simulink model "cubesat_alg_dev_env"  (R2022a)
settings: Solver=FixedStepAuto  StartTime=0.0  StopTime=604800  FixedStep=0.5  MaxStep=1  MinStep=0.01  RelTol=1e-3
undefined symbols (not defined in the file or in its folder): km, s, WMM2020
libraries: aerolibutil x5, matrix_library x3, simulink_extras x1, vrlib x1, aerolibcelestial x1, aerolibgravity2 x1
settings Model: SimulationMode=accelerator  Creator=samuel  LastModifiedBy=samuel

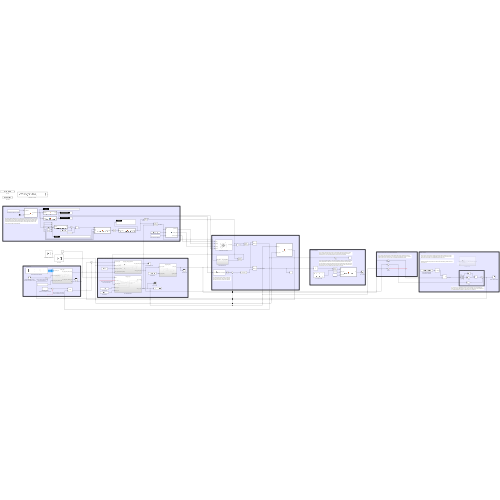
[thumbnail: Simulink's stored preview of the top-level diagram]
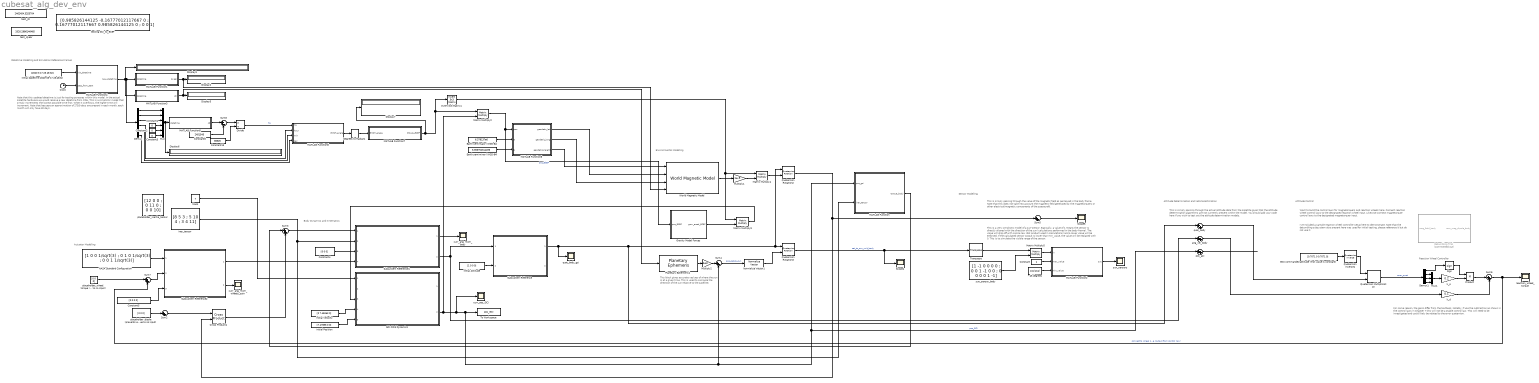
== system cubesat_alg_dev_env ==
  note: This block gives accurate vaslues of where the sun is at a given time. This is used to compute the direction of the sun relative to the satellite.
  note: For some reason, the gains differ from the textbook. Notably, if use the subtraction as shown in the control laws in Chapter 7 this will not be a stable control law. This will need to be investigated and could likely be related to the error quaternion.
  note: Reaction Wheel Controller
  note: I've included a sample reaction wheel controller setup here to demonstrate. Note that the detumbling subsystem also present here was used for initial testing, please reference it but do not use it.
  note: Want to build the control laws for magnetorquers and reaction wheels here. Connect reaction wheel control laws to the designated reaction wheel input. Likewise connect magnetorquer control laws to the designated magnetorquer input.
  note: Note that this updated datetime is just for testing purposes within this model. In the actual satellite hardware we would receive a new datetime from CDH. This is a simplistic model that simply increments the lowest possible time first. When it overflows, the higher time will increment. Note that becuase an approximation of 275/9 days are present in each month, each month will only have 30 days.
  note: This is simply passing through the value of the magnetic field as perceived in the body frame. Note that this does not take into account the magnetic field generated by the magnetorquers or other electrical/magnetic components of the spacecraft.
  note: This is a very simplistic model of a sun-sensor. Basically, a value of 1 means the sensor is directly aligned with the direction of the sun (calculations performed in the body-frame). The value will drop off with cosine law (dot product used in calculations) and a lower value will be enforced. If the calculated sensor output is lower than min_value, the value will be replaced with 0. This is to simulate the visible range of the sensor.
  note: This is simply passing through the actual atittude data from the satellite given that the attitude determination algorithms are not currently present within the model. You should add your code here if you wish to test out the attitude determination models.
  note: Datetime Modelling and Simulation Reference Frames
  note: Attitude Control
  note: Actuator Modelling
  note: Attitude Determination and Vehicle Estimation
  note: Sensor Modelling
  note: Environmental Modelling
  note: Body Dynamics and Kinematics
  Clock : Clock
  Constant : Constant
  Constant1 : Constant  Value=0
  Constant13 : Constant  Value=36525
  Constant2 : Constant  Value=0
  Constant3 : Constant  Value=0
  Constant4 : Constant  Value=[0 0 0]
  Constant5 : Constant  Value=[0 0 0 0]
  Constant6 : Constant  Value=2451545
  Cross Product1 : matrix_library/Cross Product
      settings: SourceProductBaseCode=SL
  Degrees to Radians : simulink_extras/Transformations/Degrees to Radians
  Demux : Demux  Outputs=6
  Demux1 : Demux
  Detumbling Trial : Subsystem  Commented=on
  Display{2..3,5..7} (5 alike) : Display
  Divide : Product  Inputs=*/
  Earth semimajor (WGS-84) : Constant  Value=6.378137e6
  Earth semiminor (WGS-84) : Constant  Value=6.3567523142e6
  GCI COG Dynamics : Subsystem  ReferencedSubsystem=cog_dyn_gci
  Gravity Model Forces : Subsystem
  Initial Attitude : Constant  Value=[1 0 0 0]
  Initial Datetime 2020-03-17 23:48:32 : Constant  Value=[2020 3 17 23 48 32]
  Initial Position : Constant  Value=[7.178e6 0 0]
  Initial Velocity : Constant  Value=[0 7.452e3 0]
  Invert 3x3 Matrix1 : aerolibutil/Invert  3x3 Matrix
  MATLAB Function : MATLAB Function  TreatAsAtomicUnit=on
  MATLAB Function1 : MATLAB Function  TreatAsAtomicUnit=on
  MATLAB Function2 : MATLAB Function  TreatAsAtomicUnit=on
  MATLAB Function3 : MATLAB Function  TreatAsAtomicUnit=on
  MATLAB Function4 : MATLAB Function  TreatAsAtomicUnit=on
  MATLAB Function5 : MATLAB Function  TreatAsAtomicUnit=on
  MATLAB Function6 : MATLAB Function  TreatAsAtomicUnit=on
  MATLAB Function7 : MATLAB Function  TreatAsAtomicUnit=on
  MATLAB Function8 : MATLAB Function  TreatAsAtomicUnit=on
  Mass : Constant  Value=7
  Matrix Multiply{2..5} (4 alike) : Product  Multiplication=Matrix(*)
  Multiply1 : Gain  Gain=1e-9
  Multiply2 : Gain  Gain=1e3
  Mux : Mux  Inputs=6
  Mux1 : Mux  Inputs=3
  NASA Standard Configuration : Constant  Value=[1 0 0 1/sqrt(3) ; 0 1 0 1/sqrt(3) ; 0 0 1 1/sqrt(3)]
  Normalize Vector1 : vrlib/Utilities/Normalize Vector  maxzero=0
  Planetary Ephemeris1 : aerolibcelestial/Planetary Ephemeris  kmflag=km,km/s  epochflag=Julian date  de=DE405  nCenter=Earth  nTarget=Sun  errorflag=Error  velflag=off
      settings: SourceProductBaseCode=AE
  Product : Product
  Quaternion Inverse1 : aerolibutil/Quaternion Inverse
  Quaternion Multiplication : aerolibutil/Quaternion Multiplication
  Quaternion Rotation2 : aerolibutil/Quaternion Rotation
  Quaternion Rotation3 : aerolibutil/Quaternion Rotation
  Scope4 : Scope
  Scope5 : Scope
  Sign : Signum
  Subsystem Reference : Subsystem  ReferencedSubsystem=quat_kin_body
  Subsystem Reference1 : Subsystem  ReferencedSubsystem=quat_dyn_body_w_wheels
  Subsystem Reference2 : Subsystem  ReferencedSubsystem=wheel_dyn
  Sum{2..3,5..7} (5 alike) : Sum  Inputs=|++
  Sum4 : Sum  Inputs=|+-
  Sum8 : Sum  Inputs=|+-
  To Workspace : ToWorkspace  VariableName=pos_GCI  SampleTime=-1
  Transpose : matrix_library/Transpose
      settings: SourceProductBaseCode=SL
  World Magnetic Model : aerolibgravity2/World Magnetic Model  model=WMM2020 (2020-2025)  customFile='WMM2020.COF'  units=Metric (MKS)  time_in=on  month=January  day=1  year=2020  action=Error  h_out=off  dec_out=off  inc_out=off  ti_out=off
      settings: SourceProductBaseCode=AE
  ang_vel_body : Sum  Inputs=|++
  curr_ang_mom_body : Scope
  curr_ang_mom_wheels_spin : Scope
  curr_pos_GCI : Scope
  iner_tensor : Constant  Value=[8 5 3 ; 5 10 4 ; 3 4 11]
  k_d : Gain  Gain=0.1
  k_p : Gain  Gain=0.2
  placeholder_dipole (prevents errors due to no input) : Constant  Value=[0 0 0]
  placeholder_inertia_tensor : Constant  Value=[12 0 0 ; 0 11 0 ; 0 0 10]
  placeholder_wheel_torque (prevents errors due to no input) : Constant  Value=[0 0 0]
  pos_gci : Sum  Inputs=|++
  quat_body : Sum  Inputs=|++
  quat_body_gci : Scope
  reaction_wheel_torque : Scope
  sun_sensor_body : Constant  Value=[1 -1 0 0 0 0 ; 0 0 1 -1 0 0 ; 0 0 0 0 1 -1]
  sun_sensors : Scope
  test commanded attitude (first value is constant) : Constant  Value=[0.7071 0 0.7071 0]
  test_JD : Constant  Value=2462454.3253704
  test_dyear : Constant  Value=2020.2986146465
  testing GCI_to_ECEF : Constant  Value=[0.985826144125 -0.16777012117667 0 ; 0.16777012117667 0.985826144125 0 ; 0 0 1]
  ~45 degrees : Constant  Value=cos(pi/4)
  wires:
  NASA Standard Configuration/1 -> Subsystem Reference2/1
  Initial Attitude/1 -> Subsystem Reference/2
  Constant5/1 -> Subsystem Reference2/3
  Mass/1 -> GCI COG Dynamics/1
  Initial Velocity/1 -> GCI COG Dynamics/4
  Initial Position/1 -> GCI COG Dynamics/5
  GCI COG Dynamics/2 -> To Workspace/1, pos_gci/1, MATLAB Function/1(pos_gci), Sum4/2, curr_pos_GCI/1, Matrix Multiply2/2  "pos_GCI"
  Sum7/1 -> Subsystem Reference2/2
  Subsystem Reference2/2 -> curr_ang_mom_wheels_spin/1
  Matrix Multiply2/1 -> MATLAB Function8/1(pos), Gravity Model Forces/1(pos_ECEF)  "pos_ECEF"
  MATLAB Function8/1(geodetic_lat) -> World Magnetic Model/2
  MATLAB Function8/2(geodetic_long) -> World Magnetic Model/3
  MATLAB Function8/3(geodetic_height) -> World Magnetic Model/1
  Gravity Model Forces/1(grav_accel_ECEF) -> Matrix Multiply3/2
  Invert 3x3 Matrix1/1 -> Matrix Multiply4/1, Matrix Multiply3/1
  Matrix Multiply3/1 -> GCI COG Dynamics/3
  iner_tensor/1 -> MATLAB Function/2(iner_tensor), Subsystem Reference1/2
  Constant4/1 -> Subsystem Reference1/3
  Subsystem Reference2/1 -> Subsystem Reference1/4
  Subsystem Reference1/1 -> curr_ang_mom_body/1
  Subsystem Reference1/2 -> ang_vel_body/1, Subsystem Reference/1
  World Magnetic Model/1 -> Multiply1/1
  Multiply1/1 -> Matrix Multiply4/2
  Matrix Multiply4/1 -> Quaternion Rotation2/2
  Subsystem Reference/1 -> Quaternion Rotation2/1, Quaternion Rotation3/1, quat_body/1, quat_body_gci/1
  placeholder_dipole (prevents errors due to no input)/1 -> Sum2/1
  ? -> Sum2/2  "connect to magnetic control dipole (output from magnetorquer model)"
  Quaternion Rotation2/1 -> Cross Product1/2, Sum5/1
  Sum2/1 -> Cross Product1/1
  Sum3/1 -> Subsystem Reference1/1
  Cross Product1/1 -> Sum3/2
  MATLAB Function/1(torque_body) -> Sum3/1
  Planetary Ephemeris1/1 -> Multiply2/1
  Normalize Vector1/1 -> Quaternion Rotation3/2
  Multiply2/1 -> Sum4/1
  Sum4/1 -> Normalize Vector1/1  "pos_sat_to_sun"
  sun_sensor_body/1 -> Matrix Multiply5/2
  Quaternion Rotation3/1 -> Scope4/1, Transpose/1  "sat_to_sun_unit_body"
  Transpose/1 -> Matrix Multiply5/1
  Sum5/1 -> Scope5/1
  Sum6/1 -> reaction_wheel_torque/1, Sum7/2  "connect to wheel control torque (output from control law)"
  placeholder_wheel_torque (prevents errors due to no input)/1 -> Sum7/1
  Matrix Multiply5/1 -> MATLAB Function2/1(in)
  Constant/1 -> MATLAB Function2/2(max_value)
  ~45 degrees/1 -> MATLAB Function2/3(min_value)
  MATLAB Function2/1(out) -> sun_sensors/1
  Clock/1 -> MATLAB Function4/2(secs_from_start)
  Initial Datetime 2020-03-17 23:48:32/1 -> MATLAB Function4/1(init_datetime)
  MATLAB Function4/1(new_datetime) -> Demux/1, MATLAB Function1/1(datetime), MATLAB Function3/1(datetime), Display3/1
  Demux/1 -> Mux/1
  Demux/2 -> Mux/2
  Demux/3 -> Mux/3
  Constant1/1 -> Mux/4
  Constant2/1 -> Mux/5
  Constant3/1 -> Mux/6
  Mux/1 -> Display6/1, MATLAB Function5/1(datetime)
  MATLAB Function5/1(JD) -> Sum8/1
  Constant6/1 -> Sum8/2
  Sum8/1 -> Divide/1
  Constant13/1 -> Divide/2
  Divide/1 -> MATLAB Function6/1(T0)  "T0"
  Demux/4 -> MATLAB Function6/2(hour)
  Demux/5 -> MATLAB Function6/3(min)
  Demux/6 -> MATLAB Function6/4(sec)
  MATLAB Function6/1(GMST_angle) -> Degrees to Radians/1
  Degrees to Radians/1 -> MATLAB Function7/1(GMST_angle)
  MATLAB Function7/1(GCI_to_ECEF) -> Matrix Multiply2/1, Invert 3x3 Matrix1/1, Display7/1
  MATLAB Function3/1(JD) -> Planetary Ephemeris1/1, Display5/1
  MATLAB Function1/1(dyear) -> World Magnetic Model/4, Display2/1
  ang_vel_body/1 -> k_d/1
  pos_gci/1 -> ?
  ? -> GCI COG Dynamics/2  "want to connect orbital disturbance forces to this block here"
  Demux1/2 -> Mux1/1
  Demux1/3 -> Mux1/2
  Demux1/4 -> Mux1/3
  Demux1/1 -> Sign/1
  Mux1/1 -> k_p/1
  k_p/1 -> Product/2
  Sign/1 -> Product/1
  Product/1 -> Sum6/1
  k_d/1 -> Sum6/2
  Quaternion Multiplication/1 -> Demux1/1  "error_quat"
  test commanded attitude (first value is constant)/1 -> Quaternion Inverse1/1
  Quaternion Inverse1/1 -> Quaternion Multiplication/1
  quat_body/1 -> Quaternion Multiplication/2
  Earth semiminor (WGS-84)/1 -> MATLAB Function8/3(b)
  Earth semimajor (WGS-84)/1 -> MATLAB Function8/2(a)

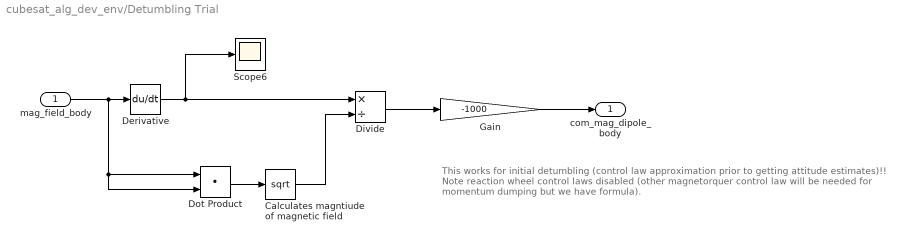
== system cubesat_alg_dev_env/Detumbling Trial ==
  note: This works for initial detumbling (control law approximation prior to getting attitude estimates)!! Note reaction wheel control laws disabled (other magnetorquer control law will be needed for momentum dumping but we have formula).
  mag_field_body : Inport
  Calculates magntiude of magnetic field : Sqrt
  Derivative : Derivative
  Divide : Product  Inputs=*/
  Dot Product : DotProduct  OutDataTypeStr=Inherit: Inherit via internal rule
  Gain : Gain  Gain=-1000
  Scope6 : Scope
  com_mag_dipole_body : Outport
  wires:
  Calculates magntiude of magnetic field/1 -> Divide/2
  Gain/1 -> com_mag_dipole_body/1
  Dot Product/1 -> Calculates magntiude of magnetic field/1
  Divide/1 -> Gain/1
  mag_field_body/1 -> Derivative/1, Dot Product/2, Dot Product/1
  Derivative/1 -> Divide/1, Scope6/1

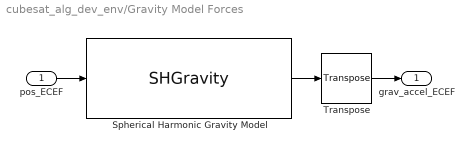
== system cubesat_alg_dev_env/Gravity Model Forces ==
  pos_ECEF : Inport
  Spherical Harmonic Gravity Model : SHGravity
  Transpose : matrix_library/Transpose
      settings: SourceProductBaseCode=SL
  grav_accel_ECEF : Outport
  wires:
  Spherical Harmonic Gravity Model/1 -> Transpose/1
  Transpose/1 -> grav_accel_ECEF/1
  pos_ECEF/1 -> Spherical Harmonic Gravity Model/1

== matlab function cubesat_alg_dev_env/MATLAB Function ==
  data: pos_gci input; torque_body output; iner_tensor input
function torque_body  = grav_grad_torque(pos_gci, iner_tensor)
    % mass of earth, grav constant
    m_e = 5.97219e24;
    G = 6.67430e-11;

    % grav param
    u = G*m_e;

    radius = norm(pos_gci);
    nadir_vec = -normalize(pos_gci);
    torque_body = cross(3*u/radius^3*nadir_vec, ...
        iner_tensor*nadir_vec);

== matlab function cubesat_alg_dev_env/MATLAB Function1 ==
  data: datetime input; dyear output
function dyear = dyear_from_datetime(datetime)

    % the datetime format is provided as a 6 value array
    % year, month, day, hour, minute, second

    % sequentially builds the decimal year

    % potentially we may want to use /61 for leap second days but this is
    % likely fine as our simulation just needs to perform regular datetime
    % updates for simple testing

    tot_mins = datetime(5) + datetime(6) / 60;
    tot_hours = datetime(4) + tot_mins / 60;
    tot_days = datetime(3) + tot_hours / 24;
    tot_months = datetime(2) + tot_days / (275/9); % average days in month across year
    tot_years = datetime(1) + tot_months / 12;

    dyear = tot_years;

== matlab function cubesat_alg_dev_env/MATLAB Function2 ==
  data: in input; out output; max_value input; min_value input
function out = zero_out_out_of_range(in, max_value, min_value)
    out = in;

    for i = 1:length(in)
        if out(i) < min_value || out(i) > max_value
            out(i) = 0;
        end
    end

== matlab function cubesat_alg_dev_env/MATLAB Function3 ==
  data: datetime input; JD output
function JD = calc_JD_from_datetime(datetime)

% the datetime format is provided as a 6 value array
% year, month, day, hour, minute, second

% calculates the Julian date (JD) from the datetime
JD = 1721013.5 + 367*datetime(1) - floor(7/4*(datetime(1) + ...
    floor((datetime(2) + 9)/12))) + floor(275/9*datetime(2)) + ...
    datetime(3) + (60*datetime(4) + datetime(5) + datetime(6)/60)/1440;

% note that seconds should be /61 for leap days but since we are using a
% testing environment we do not need to worry about this

% presumably in the navigation system of the actual satellite we may also
% not need to consider this as it would introduce a negligible error or we
% may need to have some special protocol with CDH to figure out a system

== matlab function cubesat_alg_dev_env/MATLAB Function4 ==
  data: init_datetime input; new_datetime output; secs_from_start input
function new_datetime  = datetime_upd(init_datetime, secs_from_start)

% the datetime format is provided as a 6 value array
% year, month, day, hour, minute, second

% initializes new datetime array
new_datetime = zeros(1, 6);

% adds the seconds from start of simulation to seconds
new_datetime(6) = init_datetime(6) + secs_from_start;

% computes the new seconds and minutes with carry over
new_datetime(5) = init_datetime(5) + floor(new_datetime(6) / 60);
new_datetime(6) = mod(new_datetime(6), 60);

% computes the new minutes and hours with carry over
new_datetime(4) = init_datetime(4) + floor(new_datetime(5) / 60);
new_datetime(5) = mod(new_datetime(5), 60);

% computes the new hours and days with carry over
new_datetime(3) = init_datetime(3) + floor(new_datetime(4) / 24);
new_datetime(4) = mod(new_datetime(4), 24);

% computes the new days and months with carry over
new_datetime(2) = init_datetime(2) + floor(new_datetime(3) / (275/9));

% NOTE: the floor here is specifically needed to prevent a recurring
% decimal from occurring here due to using an average number of days per
% month of 275/9 (this also caps days in a month to 30)
new_datetime(3) = floor(mod(new_datetime(3), (275/9)));

% computes the new months and years with carry over

% for calculations, shifts first month to 0
new_datetime(2) = new_datetime(2) - 1;

new_datetime(1) = init_datetime(1) + floor(new_datetime(2) / 12);

% done with calculations, restores first month to 1
new_datetime(2) = mod(new_datetime(2), 12) + 1;

end

== matlab function cubesat_alg_dev_env/MATLAB Function5 ==
  data: datetime input; JD output
function JD = calc_JD_from_datetime(datetime)

% the datetime format is provided as a 6 value array
% year, month, day, hour, minute, second

% calculates the Julian date (JD) from the datetime
JD = 1721013.5 + 367*datetime(1) - floor(7/4*(datetime(1) + ...
    floor((datetime(2) + 9)/12))) + floor(275/9*datetime(2)) + ...
    datetime(3) + (60*datetime(4) + datetime(5) + datetime(6)/60)/1440;

% note that seconds should be /61 for leap days but since we are using a
% testing environment we do not need to worry about this

% presumably in the navigation system of the actual satellite we may also
% not need to consider this as it would introduce a negligible error or we
% may need to have some special protocol with CDH to figure out a system

== matlab function cubesat_alg_dev_env/MATLAB Function6 ==
  data: T0 input; GMST_angle output; hour input; min input; sec input
function GMST_angle = calc_GMST_angle_from_T0(T0, hour, min, sec)

% calculates GMST_angle in units of seconds (longitudinal seconds)
GMST_angle = 24110.54841 + 8640184.812866 * T0 + 0.093104 * T0^2 ...
    - 6.2e-6 * T0^3 + 1.002737909350795 * (3600*hour + 60*min + sec);

% reduces to range of 0-86400
GMST_angle = mod(GMST_angle, 86400);

% converts to degrees (there are 240 longitudinal seconds in a degree)
GMST_angle = GMST_angle / 240;

== matlab function cubesat_alg_dev_env/MATLAB Function7 ==
  data: GMST_angle input; GCI_to_ECEF output
function GCI_to_ECEF = calc_GCI_to_ECEF_from_GMST_angle(GMST_angle)

% calculates the transformation matrix from GCI to ECEF
GCI_to_ECEF = [cos(GMST_angle) sin(GMST_angle) 0 ; ...
    -sin(GMST_angle) cos(GMST_angle) 0 ; 0 0 1];

== matlab function cubesat_alg_dev_env/MATLAB Function8 ==
  data: pos input; geodetic_lat output; a input; b input; geodetic_long output; geodetic_height output
function [geodetic_lat, geodetic_long, geodetic_height] = ...
    ECEF_coords_to_geodetic(pos, a, b)

    % converts from ECEF coordinates to geodetic coordinates

    x = pos(1);
    y = pos(2);
    z = pos(3);

    e2 = 1 - b^2 / a^2;
    eps2 = a^2 / b^2 - 1;
    rho = sqrt(x^2 + y^2);

    p = abs(z)/eps2;
    s = rho^2/(e2*eps2);
    q = p^2 - b^2 + s;

    u = p/sqrt(q);
    v = b^2*u^2/q;
    P=27*v*s/q;
    Q=(sqrt(P+1) + sqrt(P))^(2/3);

    t=(1+Q+1/Q)/6;
    c=sqrt(u^2-1+2*t);
    w=(c-u)/2;

    d=sign(z)*sqrt(q)*(w+sqrt(t^2+v)-u*w-t/2-1/4);

    N = a*sqrt(1+eps2*d^2/b^2);
    lat = asin((eps2+1)*(d/N));
    
    h = rho*cos(lat)+z*sin(lat)-a^2/N;
    long = atan2(y, x);

    % converts from rad to deg
    geodetic_lat = rad2deg(lat);
    geodetic_long = rad2deg(long);

    geodetic_height = h;
